simulink model "dcp_forPic"  (R2015b)
settings: Solver=ode45  SolverMode=SingleTasking  StartTime=0.0  StopTime=10.0  RelTol=1e-3
undefined symbols (not defined in the file): cars1, cars2, cars3, const, mat, numCars, param
libraries: CarMaker4SL x10, simulink x1
(part 2 of 2)

== system dcp_forPic/CarMaker/IPG Vehicle/CarAndTrailer/Trailer/CreateBus Vhcl.Wheel.FR ==
  In1 : Inport
  Bus Creator3 : BusCreator  Inputs=14
  Demux3 : Demux  Outputs=14
  Out1 : Outport
  wires:
  Demux3/14 -> Bus Creator3/14  "Vhcl Wheel FR Trq_WhlBearing"
  Demux3/13 -> Bus Creator3/13  "Vhcl Wheel FR Trq_T2W"
  Demux3/12 -> Bus Creator3/12  "Vhcl Wheel FR SideSlip"
  Demux3/11 -> Bus Creator3/11  "Vhcl Wheel FR LongSlip"
  Demux3/10 -> Bus Creator3/10  "Vhcl Wheel FR vBelt"
  Demux3/9 -> Bus Creator3/9  "Vhcl Wheel FR Fz"
  Demux3/8 -> Bus Creator3/8  "Vhcl Wheel FR Fy"
  Demux3/7 -> Bus Creator3/7  "Vhcl Wheel FR Fx"
  Demux3/6 -> Bus Creator3/6  "Vhcl Wheel FR r_zxy z"
  Demux3/5 -> Bus Creator3/5  "Vhcl Wheel FR r_zxy y"
  Demux3/4 -> Bus Creator3/4  "Vhcl Wheel FR r_zxy x"
  Demux3/3 -> Bus Creator3/3  "Vhcl Wheel FR t z"
  Demux3/2 -> Bus Creator3/2  "Vhcl Wheel FR t y"
  In1/1 -> Demux3/1
  Bus Creator3/1 -> Out1/1
  Demux3/1 -> Bus Creator3/1  "Vhcl Wheel FR t x"

== system dcp_forPic/CarMaker/IPG Vehicle/CarAndTrailer/Trailer/CreateBus Vhcl.Wheel.RL ==
  In1 : Inport
  Bus Creator3 : BusCreator  Inputs=14
  Demux3 : Demux  Outputs=14
  Out1 : Outport
  wires:
  Demux3/14 -> Bus Creator3/14  "Vhcl Wheel RL Trq_WhlBearing"
  Demux3/13 -> Bus Creator3/13  "Vhcl Wheel RL Trq_T2W"
  Demux3/12 -> Bus Creator3/12  "Vhcl Wheel RL SideSlip"
  Demux3/11 -> Bus Creator3/11  "Vhcl Wheel RL LongSlip"
  Demux3/10 -> Bus Creator3/10  "Vhcl Wheel RL vBelt"
  Demux3/9 -> Bus Creator3/9  "Vhcl Wheel RL Fz"
  Demux3/8 -> Bus Creator3/8  "Vhcl Wheel RL Fy"
  Demux3/7 -> Bus Creator3/7  "Vhcl Wheel RL Fx"
  Demux3/6 -> Bus Creator3/6  "Vhcl Wheel RL r_zxy z"
  Demux3/5 -> Bus Creator3/5  "Vhcl Wheel RL r_zxy y"
  Demux3/4 -> Bus Creator3/4  "Vhcl Wheel RL r_zxy x"
  Demux3/3 -> Bus Creator3/3  "Vhcl Wheel RL t z"
  Demux3/2 -> Bus Creator3/2  "Vhcl Wheel RL t y"
  In1/1 -> Demux3/1
  Bus Creator3/1 -> Out1/1
  Demux3/1 -> Bus Creator3/1  "Vhcl Wheel RL t x"

== system dcp_forPic/CarMaker/IPG Vehicle/CarAndTrailer/Trailer/CreateBus Vhcl.Wheel.RR ==
  In1 : Inport
  Bus Creator3 : BusCreator  Inputs=14
  Demux3 : Demux  Outputs=14
  Out1 : Outport
  wires:
  Demux3/14 -> Bus Creator3/14  "Vhcl Wheel RR Trq_WhlBearing"
  Demux3/13 -> Bus Creator3/13  "Vhcl Wheel RR Trq_T2W"
  Demux3/12 -> Bus Creator3/12  "Vhcl Wheel RR SideSlip"
  Demux3/11 -> Bus Creator3/11  "Vhcl Wheel RR LongSlip"
  Demux3/10 -> Bus Creator3/10  "Vhcl Wheel RR vBelt"
  Demux3/9 -> Bus Creator3/9  "Vhcl Wheel RR Fz"
  Demux3/8 -> Bus Creator3/8  "Vhcl Wheel RR Fy"
  Demux3/7 -> Bus Creator3/7  "Vhcl Wheel RR Fx"
  Demux3/6 -> Bus Creator3/6  "Vhcl Wheel RR r_zxy z"
  Demux3/5 -> Bus Creator3/5  "Vhcl Wheel RR r_zxy y"
  Demux3/4 -> Bus Creator3/4  "Vhcl Wheel RR r_zxy x"
  Demux3/3 -> Bus Creator3/3  "Vhcl Wheel RR t z"
  Demux3/2 -> Bus Creator3/2  "Vhcl Wheel RR t y"
  In1/1 -> Demux3/1
  Bus Creator3/1 -> Out1/1
  Demux3/1 -> Bus Creator3/1  "Vhcl Wheel RR t x"

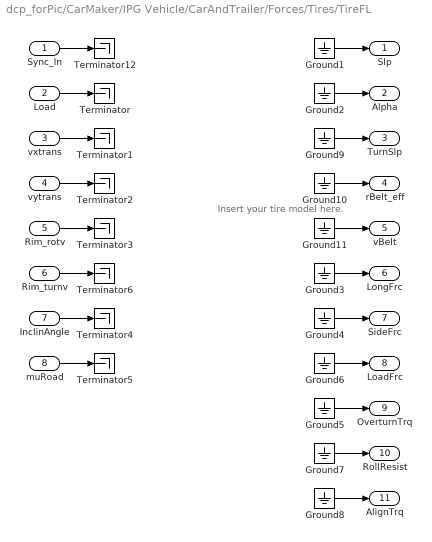
== system dcp_forPic/CarMaker/IPG Vehicle/CarAndTrailer/Forces/Tires/TireFL ==
  note: Insert your tire model here.
  Sync_In : Inport
  Load : Inport  Port=2
  vxtrans : Inport  Port=3
  vytrans : Inport  Port=4
  Rim_rotv : Inport  Port=5
  Rim_turnv : Inport  Port=6
  InclinAngle : Inport  Port=7
  muRoad : Inport  Port=8
  Ground{1..11} (11 alike) : Ground
  Terminator{,1..6,12} (8 alike) : Terminator
  Slp : Outport
  Alpha : Outport  Port=2
  TurnSlp : Outport  Port=3
  rBelt_eff : Outport  Port=4
  vBelt : Outport  Port=5
  LongFrc : Outport  Port=6
  SideFrc : Outport  Port=7
  LoadFrc : Outport  Port=8
  OverturnTrq : Outport  Port=9
  RollResist : Outport  Port=10
  AlignTrq : Outport  Port=11
  wires:
  Ground11/1 -> vBelt/1
  Ground10/1 -> rBelt_eff/1
  Ground9/1 -> TurnSlp/1
  Rim_turnv/1 -> Terminator6/1
  Sync_In/1 -> Terminator12/1
  Ground2/1 -> Alpha/1
  Ground3/1 -> LongFrc/1
  Ground4/1 -> SideFrc/1
  Ground5/1 -> OverturnTrq/1
  vxtrans/1 -> Terminator1/1
  vytrans/1 -> Terminator2/1
  Rim_rotv/1 -> Terminator3/1
  InclinAngle/1 -> Terminator4/1
  muRoad/1 -> Terminator5/1
  Load/1 -> Terminator/1
  Ground1/1 -> Slp/1
  Ground6/1 -> LoadFrc/1
  Ground7/1 -> RollResist/1
  Ground8/1 -> AlignTrq/1

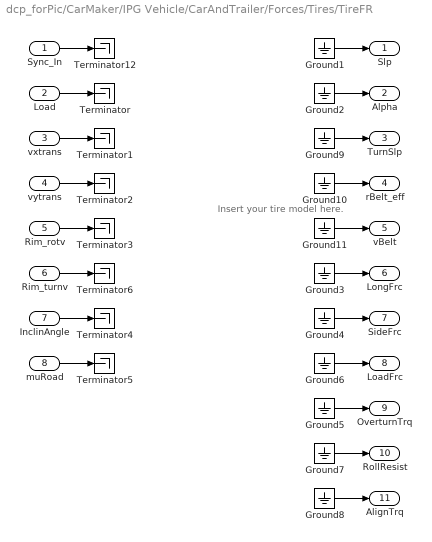
== system dcp_forPic/CarMaker/IPG Vehicle/CarAndTrailer/Forces/Tires/TireFR ==
  note: Insert your tire model here.
  Sync_In : Inport
  Load : Inport  Port=2
  vxtrans : Inport  Port=3
  vytrans : Inport  Port=4
  Rim_rotv : Inport  Port=5
  Rim_turnv : Inport  Port=6
  InclinAngle : Inport  Port=7
  muRoad : Inport  Port=8
  Ground{1..11} (11 alike) : Ground
  Terminator{,1..6,12} (8 alike) : Terminator
  Slp : Outport
  Alpha : Outport  Port=2
  TurnSlp : Outport  Port=3
  rBelt_eff : Outport  Port=4
  vBelt : Outport  Port=5
  LongFrc : Outport  Port=6
  SideFrc : Outport  Port=7
  LoadFrc : Outport  Port=8
  OverturnTrq : Outport  Port=9
  RollResist : Outport  Port=10
  AlignTrq : Outport  Port=11
  wires:
  Ground11/1 -> vBelt/1
  Ground10/1 -> rBelt_eff/1
  Ground9/1 -> TurnSlp/1
  Rim_turnv/1 -> Terminator6/1
  Sync_In/1 -> Terminator12/1
  Ground2/1 -> Alpha/1
  Ground3/1 -> LongFrc/1
  Ground4/1 -> SideFrc/1
  Ground5/1 -> OverturnTrq/1
  vxtrans/1 -> Terminator1/1
  vytrans/1 -> Terminator2/1
  Rim_rotv/1 -> Terminator3/1
  InclinAngle/1 -> Terminator4/1
  muRoad/1 -> Terminator5/1
  Load/1 -> Terminator/1
  Ground1/1 -> Slp/1
  Ground6/1 -> LoadFrc/1
  Ground7/1 -> RollResist/1
  Ground8/1 -> AlignTrq/1

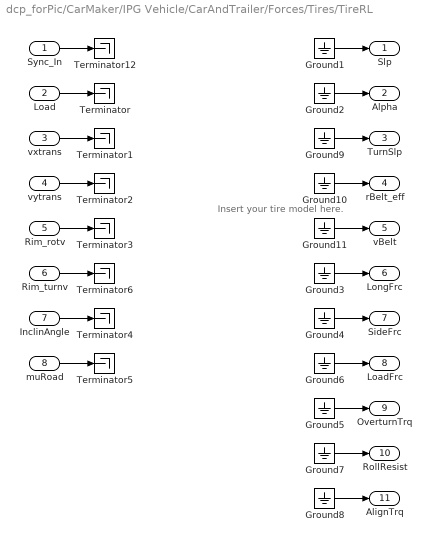
== system dcp_forPic/CarMaker/IPG Vehicle/CarAndTrailer/Forces/Tires/TireRL ==
  note: Insert your tire model here.
  Sync_In : Inport
  Load : Inport  Port=2
  vxtrans : Inport  Port=3
  vytrans : Inport  Port=4
  Rim_rotv : Inport  Port=5
  Rim_turnv : Inport  Port=6
  InclinAngle : Inport  Port=7
  muRoad : Inport  Port=8
  Ground{1..11} (11 alike) : Ground
  Terminator{,1..6,12} (8 alike) : Terminator
  Slp : Outport
  Alpha : Outport  Port=2
  TurnSlp : Outport  Port=3
  rBelt_eff : Outport  Port=4
  vBelt : Outport  Port=5
  LongFrc : Outport  Port=6
  SideFrc : Outport  Port=7
  LoadFrc : Outport  Port=8
  OverturnTrq : Outport  Port=9
  RollResist : Outport  Port=10
  AlignTrq : Outport  Port=11
  wires:
  Ground11/1 -> vBelt/1
  Ground10/1 -> rBelt_eff/1
  Ground9/1 -> TurnSlp/1
  Rim_turnv/1 -> Terminator6/1
  Sync_In/1 -> Terminator12/1
  Ground2/1 -> Alpha/1
  Ground3/1 -> LongFrc/1
  Ground4/1 -> SideFrc/1
  Ground5/1 -> OverturnTrq/1
  vxtrans/1 -> Terminator1/1
  vytrans/1 -> Terminator2/1
  Rim_rotv/1 -> Terminator3/1
  InclinAngle/1 -> Terminator4/1
  muRoad/1 -> Terminator5/1
  Load/1 -> Terminator/1
  Ground1/1 -> Slp/1
  Ground6/1 -> LoadFrc/1
  Ground7/1 -> RollResist/1
  Ground8/1 -> AlignTrq/1

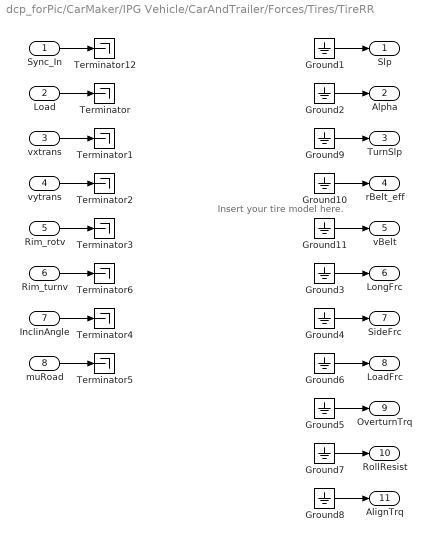
== system dcp_forPic/CarMaker/IPG Vehicle/CarAndTrailer/Forces/Tires/TireRR ==
  note: Insert your tire model here.
  Sync_In : Inport
  Load : Inport  Port=2
  vxtrans : Inport  Port=3
  vytrans : Inport  Port=4
  Rim_rotv : Inport  Port=5
  Rim_turnv : Inport  Port=6
  InclinAngle : Inport  Port=7
  muRoad : Inport  Port=8
  Ground{1..11} (11 alike) : Ground
  Terminator{,1..6,12} (8 alike) : Terminator
  Slp : Outport
  Alpha : Outport  Port=2
  TurnSlp : Outport  Port=3
  rBelt_eff : Outport  Port=4
  vBelt : Outport  Port=5
  LongFrc : Outport  Port=6
  SideFrc : Outport  Port=7
  LoadFrc : Outport  Port=8
  OverturnTrq : Outport  Port=9
  RollResist : Outport  Port=10
  AlignTrq : Outport  Port=11
  wires:
  Ground11/1 -> vBelt/1
  Ground10/1 -> rBelt_eff/1
  Ground9/1 -> TurnSlp/1
  Rim_turnv/1 -> Terminator6/1
  Sync_In/1 -> Terminator12/1
  Ground2/1 -> Alpha/1
  Ground3/1 -> LongFrc/1
  Ground4/1 -> SideFrc/1
  Ground5/1 -> OverturnTrq/1
  vxtrans/1 -> Terminator1/1
  vytrans/1 -> Terminator2/1
  Rim_rotv/1 -> Terminator3/1
  InclinAngle/1 -> Terminator4/1
  muRoad/1 -> Terminator5/1
  Load/1 -> Terminator/1
  Ground1/1 -> Slp/1
  Ground6/1 -> LoadFrc/1
  Ground7/1 -> RollResist/1
  Ground8/1 -> AlignTrq/1

== matlab function dcp_forPic/###Recovered Stateflow Charts###/CarMaker_VehicleControl_MATLAB Function2_repaired_1 ==
  data: longAcc output; param parameter; const parameter; mat parameter; cars1 parameter; cars2 parameter; cars3 parameter; numCars parameter; dist2Int input; uk input; upk input; time input; velocity input; uk1 output; upk1 output; exflag output
function [longAcc,uk1,upk1,exflag]   = MPC (param,const,mat,cars1,cars2,cars3,numCars,dist2Int,uk,upk,time,velocity)  %#codegen

coder.extrinsic('quadprog');
exflag = zeros(1,1,'double');

A = mat.A; 
B = mat.B; 
C = mat.C'; 
Q = mat.Q;

% parameter data
contR = param.contrRadius;
critZ = param.critZone;
w = [param.weights];
ds = param.sampling;
tdiff = param.timediff;

% cars = struct;

refVel = zeros(1,3);
meanVel = zeros(1,3);

refVel(1) = cars1.refVel;
refVel(2) = cars2.refVel;
refVel(3) = cars3.refVel; 

meanVel(1) = cars1.meanVel;
meanVel(2) = cars2.meanVel;
meanVel(3) = cars3.meanVel;


xk = zeros(2,3);

xk(:,1) = [time; 1/velocity(1)];
xk(:,2) = [time; 1/velocity(2)];
xk(:,3) = [time; 1/velocity(3)];

longAcc = zeros(3,1);
uk1 = zeros(3,1);
upk1 = zeros(3,1);
No = 2*contR + critZ; % total prediction horizon

% Constraints
amax = const.amax; amin = const.amin ;
vmax = const.vmax ; vmin = const.vmin ;

% N = 2*contR + critZ + (car(j).dist2Int - contR) = contR+critZ+car(j).dist2Int

% Prediction horizon for each cars
N = contR+critZ+dist2Int;
N(N < 0 | N > No) = 0; % The car have to be inside the control horizon

HM11 = zeros(270,270);
HM21 = zeros(135,135);
HM31 = zeros(135,135);

Hm1 = zeros(4*135,4*135);
f1 = zeros(4*135,1);

Ha1 = zeros(2*135,2*135);
Hi1 = zeros(2*135,2*135);

Hi11 = zeros(135-1, 135);
Hi21 = zeros(135-1, 135);

Aeq1 = zeros(3*135+1,4*135);
beq1 = zeros(3*135+1,1);

Ain1 = zeros(4*135,4*135);
bin1 = zeros(4*135,1);
  

coder.varsize('HM11', [270 270], [1 1]);
coder.varsize('HM21');
coder.varsize('HM31');
coder.varsize('Hm1');
coder.varsize('f1');
coder.varsize('Ha1');
coder.varsize('Hi1');
coder.varsize('Hi11');
coder.varsize('Hi21');
coder.varsize('Aeq1');
coder.varsize('beq1');
coder.varsize('Ain1');
coder.varsize('bin1');

% coder.varsize('eye', [135 135],[1 1]);

Eye = eye(2*135);
coder.varsize('Eye');


Zeros = zeros(4*135,4*135);
coder.varsize('Zeros');

Ones = ones(4*135,4*135);
coder.varsize('Ones');

Neq = [0 0 0];
% eye(N(j)) 

% Eye(1:N(j),1:N(j))

coder.varsize('Hm',[1620 1620]);


c = [struct('HM1',HM11,'HM2',HM21,'HM3',HM31,'Hm',Hm1,'f',f1,'Ha',Ha1,...
    'Hi',Hi1,'Hi1',Hi11,'Hi2',Hi21,'Aeq',Aeq1,'beq',beq1,'Ain',Ain1,'bin',bin1),...
     struct('HM1',HM11,'HM2',HM21,'HM3',HM31,'Hm',Hm1,'f',f1,'Ha',Ha1,...
    'Hi',Hi1,'Hi1',Hi11,'Hi2',Hi21,'Aeq',Aeq1,'beq',beq1,'Ain',Ain1,'bin',bin1),...
     struct('HM1',HM11,'HM2',HM21,'HM3',HM31,'Hm',Hm1,'f',f1,'Ha',Ha1,...
    'Hi',Hi1,'Hi1',Hi11,'Hi2',Hi21,'Aeq',Aeq1,'beq',beq1,'Ain',Ain1,'bin',bin1)];

for j=1:numCars
       
    % When a car is inside the control region the car
    % will be controlled of by the MPC. The horizon is limited to the exit
    % of the control region.
    if dist2Int(j) <= contR &&  dist2Int(j) > -(contR+critZ)
        
% Hessian Matrix and f vector        

        c(j).HM1(1:2*N(j),1:2*N(j)) = kron(Eye(1:N(j),1:N(j)),2*Q*w(1)*meanVel(j)^3);  % Part J1 opt fcn 
        c(j).HM2(1:N(j),1:N(j)) = kron(Eye(1:N(j),1:N(j)),2*w(2)*meanVel(j)^5);    % Part J2 A opt fcn
        c(j).HM3(1:N(j),1:N(j)) = kron(Eye(1:N(j),1:N(j)),2*w(3)*meanVel(j)^7);    % Part J2 B opt fcn

        c(j).Hm(1:4*N(j),1:4*N(j)) = [c(j).HM1(1:2*N(j),1:2*N(j)) Zeros(1:2*N(j),1:2*N(j))
                   Zeros(1:N(j),1:2*N(j)) c(j).HM2(1:N(j),1:N(j)) Zeros(1:N(j),1:N(j))
                   Zeros(1:N(j),1:3*N(j)) c(j).HM3(1:N(j),1:N(j))];
        
        c(j).f(1:4*N(j),1) = [kron(Ones(1,1:N(j)),-2*1/refVel(j)*w(1)*meanVel(j)^3*C') Zeros(1,1:2*N(j))]'; 
        
% Equality contraints
        
        c(j).Ha(1:2*N(j),1:2*N(j)) = [Zeros(1:2,1:2*N(j)); kron(Eye(1:(N(j)-1),1:(N(j)-1)),[1 1;0 1]) Zeros(1:(N(j)-1)*2,1:2)];
        c(j).Hi(1:2*N(j),1:2*N(j)) = Eye(1:N(j)*2,1:N(j)*2);
        c(j).Hi1(1:N(j)-1,1:N(j)) = [Eye(1:N(j)-1,1:N(j)-1) Zeros(1:(N(j)-1),1)];
        c(j).Hi2(1:N(j)-1,1:N(j)) = [Zeros(1:(N(j)-1),1) Eye(1:N(j)-1,1:N(j)-1)];
              
        Neq(j) = 3*N(j) + 1; 
        c(j).Aeq(1:(3*N(j)+1),1:4*N(j)) = ([c(j).Ha(1:2*N(j),1:2*N(j))-c(j).Hi(1:2*N(j),1:2*N(j)) kron(Eye(1:N(j),1:N(j)),B) Zeros(1:2*N(j),1:N(j))    % x+ = Ax + Bu
            Zeros(1:N(j)-1,1:2*N(j)) (c(j).Hi2(1:N(j)-1,1:N(j))-c(j).Hi1(1:N(j)-1,1:N(j)))/ds c(j).Hi1(1:N(j)-1,1:N(j)) % ]);     % u'(k) = (u(k+1) - u(k))/ds
            Zeros(1,1:2*N(j)) 1 Zeros(1,1:2*N(j)-1) %]);    % u(k) = u(k-1)
            Zeros(1,1:3*N(j)) 1 Zeros(1,1:N(j)-1)]);   % up(k) = up(k-1)


        c(j).beq(1:3*N(j)+1,1) = [-A*xk(:,j) % -A*x(0)
            Zeros(1:N(j)*3-3,1)  %];
            uk(j)
            upk(j)];
                 
        
% Inequality Constraints
        c(j).Ain(1:4*N(j),1:4*N(j)) = [kron(Eye(1:N(j),1:N(j)),C') Zeros(1:N(j),1:2*N(j))  % C*x <= 1/vmin       -> (1)
            kron(Eye(1:N(j),1:N(j)),-C') Zeros(1:N(j),1:2*N(j)) % -C*x <= -1/vmax     -> (2)
            kron(Eye(1:N(j),1:N(j)),-3*amax/refVel(j)^2*C') -Eye(1:N(j),1:N(j)) Zeros(1:N(j),1:N(j)) % -> (3)
            kron(Eye(1:N(j),1:N(j)),3*amin/refVel(j)^2*C') Eye(1:N(j),1:N(j)) Zeros(1:N(j),1:N(j))]; % -> (4)

        
         c(j).bin(1:4*N(j),1) = [Ones(1:N(j),1).*1/vmin                % (1)
            Ones(1:N(j),1).*(-1/vmax)             % (2)
            Ones(1:N(j),1).*(-2*amax/refVel(j)^3)    % (3)
            Ones(1:N(j),1).*(2*amin/refVel(j)^3)];   % (4)
        
    else
        c(j).Hm = []; c(j).f = [];
        c(j).Aeq = []; c(j).beq = [];
        c(j).Ain = []; c(j).bin = [];
    end
end



% Cronologic crossing order Car 1-> Car 2 -> Car 3

ind = find(dist2Int< contR &  dist2Int > -(contR+critZ));
leni = length(ind);
% index for cars insife control region

Aeq = blkdiag(c(1).Aeq(1:Neq(1),1:4*N(1)),c(2).Aeq(1:Neq(2),1:4*N(2)),c(3).Aeq(1:Neq(3),1:4*N(3)));
coder.varsize('Aeq',[3*4*135+2, 3*4*135+2]);
n = 0;
if  leni >= 2 % if 2 or more cars is in the control region
 
if time>=19.425
    stop = 1;
end
  
    for j=1: length(ind)-1
        leave = (dist2Int(ind(j))+critZ); % index [m] for first car to leave
        enter = (dist2Int(ind(j+1))); % index [m] for next car to enter
        
        
        if min(leave,enter) >= 1
            n = n+1;
            Aeq = blkdiag(Aeq,0);            
            Aeq(end,2*leave-1 + 4*sum(N(1:(ind(j)-1)))) = -1;
            Aeq(end,2*enter-1 + 4*sum(N(1:(ind(j+1)-1)))) = 1;
            Aeq(end,4*sum(N)+n) = -1;
            

        end
    end
end

H4 = kron(Eye(1:n,1:n),2*w(4));
f4 = kron(Ones(1:n,1),-2*w(4)*tdiff);

beq4 = Zeros(1:n,1);
Ain4 = -Ones(1:n,1:n);
bin4 = Zeros(1:n,1);

coder.varsize('H4','f4','Aeq4','beq4','Ain4','bin4')
% Combined Hessian Matrix and f vector
% ----------------------
Hm = blkdiag(c(1).Hm(1:4*N(1),1:4*N(1)),c(2).Hm(1:4*N(2),1:4*N(2)),c(3).Hm(1:4*N(3),1:4*N(3)),H4);
f = vertcat(c(1).f(1:4*N(1),1),c(2).f(1:4*N(2),1),c(3).f(1:4*N(3),1),f4);

% Equality Constraints Ain*x == bin
% ----------------------

% Aeq = blkdiag(c(1).Aeq(1:Neq(1),1:4*N(1)),c(2).Aeq(1:Neq(2),1:4*N(2)),c(3).Aeq(1:Neq(3),1:4*N(3)),Aeq4);
beq = vertcat(c(1).beq(1:Neq(1),1),c(2).beq(1:Neq(2),1),c(3).beq(1:Neq(3),1),beq4);


% In-Equality Constraints Ain*x <= bin
% ----------------------
Ain = blkdiag(c(1).Ain(1:4*N(1),1:4*N(1)),c(2).Ain(1:4*N(2),1:4*N(2)),c(3).Ain(1:4*N(3),1:4*N(3)),Ain4);

bin = vertcat(c(1).bin(1:4*N(1),1),c(2).bin(1:4*N(2),1),c(3).bin(1:4*N(3),1),bin4);





    

    
    %     elseif leavInt1 >=1
    %
    %         % Ain(end,2*leave1 -1) = 1;           % Car 1 leaving at index 2*Nze1-1
    %         % Ain(end,4*pf + 2*leave2 - 1) = -1;  % Car 2 enterng at index 4*N + 2*Nzs2 - 1
    %
    %         offset = offset + 1;
    %         Ain(end,2*leavInt1 -1 + 2*offset ) = 1;           % Car 1 leaving at index 2*Nze1-1
    %         Ain(end,4*(N1+1) + 2*entInt2 - 1+ 2*offset) = -1;  % Car 2 enterng at index 4*N + 2*Nzs2 - 1
    


% Configuration quadprog
% ----------------------
coder.extrinsic('optimset');
options = optimset('Algorithm','interior-point-convex','Display','off');


% If any car is within the control region the MPC will optimize the path
% for all cars within the controlling region.
if ~isempty(Hm)
    
    x = zeros(size(Hm,2),1);
    
    
    % tic;
    [x,~,exflag] = quadprog(Hm,f,Ain,bin,Aeq,beq,[],[],[],options);
    % time = toc;
    
%     if exflag == -2
%         disp('Error: exflag == 2 ');
%     end
    
    for j=1:numCars
        
        prev = 4*sum(N(1:j-1));
        
        if N(j) > 2
            longAcc(j) = -x(2*N(j)+2 + prev)/ x(4 + prev)^3;
            uk1(j) = x(2*N(j)+2 + prev);
            upk1(j) = x(3*N(j)+2 + prev);
        else
            longAcc(j) = 0; 
            uk1(j) = 0;
            upk1(j) = 0;
        end
        
    end
    
else
    for j=1:numCars
        longAcc(j) = 0;
        uk1(j) = 0;
        upk1(j) = 0;
    end
end
